simulink model "Question9simulink_AkankshaMurali"  (R2023b)
settings: Solver=VariableStepAuto  StartTime=0.0  StopTime=10.0  RelTol=1e-3
libraries: cstblocks x6
settings Model: Creator=shash  LastModifiedBy=akank

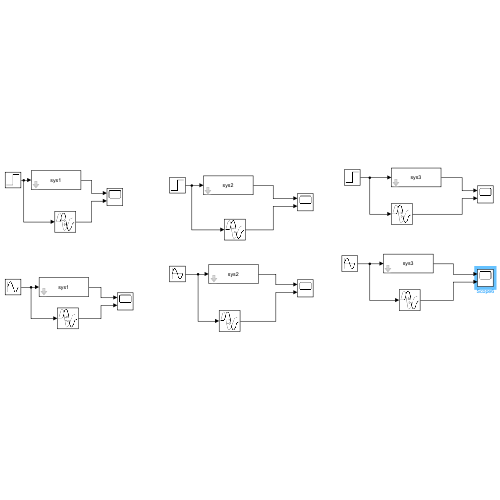
[thumbnail: Simulink's stored preview of the top-level diagram]
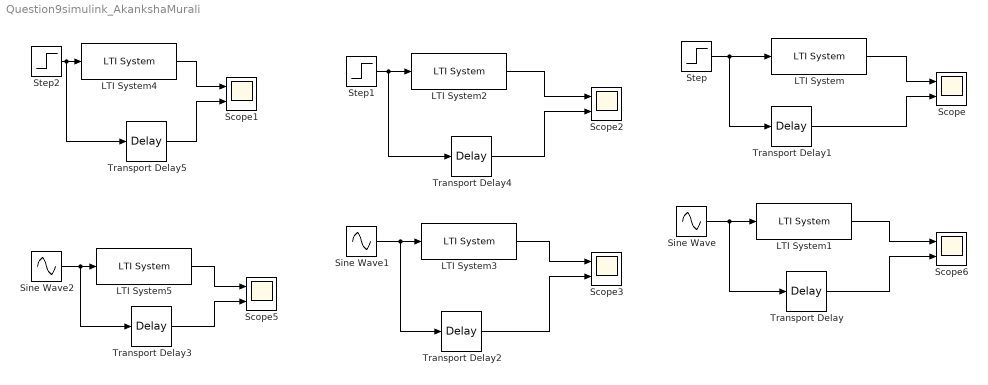
== system Question9simulink_AkankshaMurali ==
  LTI System : cstblocks/LTI System  sys=sys3  IC=[]  PadeOrder=0
  LTI System1 : cstblocks/LTI System  sys=sys3  IC=[]  PadeOrder=0
  LTI System2 : cstblocks/LTI System  sys=sys2  IC=[]  PadeOrder=0
  LTI System3 : cstblocks/LTI System  sys=sys2  IC=[]  PadeOrder=0
  LTI System4 : cstblocks/LTI System  sys=sys1  IC=[]  PadeOrder=0
  LTI System5 : cstblocks/LTI System  sys=sys1  IC=[]  PadeOrder=0
  Scope{,1..3,5..6} (6 alike) : Scope  NumInputPorts=2
  Sine Wave : Sin  Frequency=10*2*pi  SampleTime=0
  Sine Wave1 : Sin  Frequency=10*2*pi  SampleTime=0
  Sine Wave2 : Sin  Frequency=10*2*pi  SampleTime=0
  Step : Step  Time=0.1  SampleTime=0
  Step1 : Step  Time=0.1  SampleTime=0
  Step2 : Step  Time=0.1  SampleTime=0
  Transport Delay{,1..5} (6 alike) : TransportDelay  DelayTime=0.1
  wires:
  Sine Wave/1 -> Transport Delay/1, LTI System1/1
  Sine Wave2/1 -> Transport Delay3/1, LTI System5/1
  Step2/1 -> Transport Delay5/1, LTI System4/1
  Sine Wave1/1 -> Transport Delay2/1, LTI System3/1
  LTI System/1 -> Scope/1
  LTI System1/1 -> Scope6/1
  LTI System2/1 -> Scope2/1
  LTI System3/1 -> Scope3/1
  LTI System5/1 -> Scope5/1
  LTI System4/1 -> Scope1/1
  Step/1 -> Transport Delay1/1, LTI System/1
  Transport Delay/1 -> Scope6/2
  Step1/1 -> Transport Delay4/1, LTI System2/1
  Transport Delay2/1 -> Scope3/2
  Transport Delay3/1 -> Scope5/2
  Transport Delay5/1 -> Scope1/2
  Transport Delay1/1 -> Scope/2
  Transport Delay4/1 -> Scope2/2
